simulink model "Jacobian"  (R2021a)
settings: Solver=FixedStepAuto  StartTime=0.0  StopTime=5  FixedStep=0.0001  RelTol=1e-3
libraries: aerolibutil x2
settings Model: Creator=negin  LastModifiedBy=negin

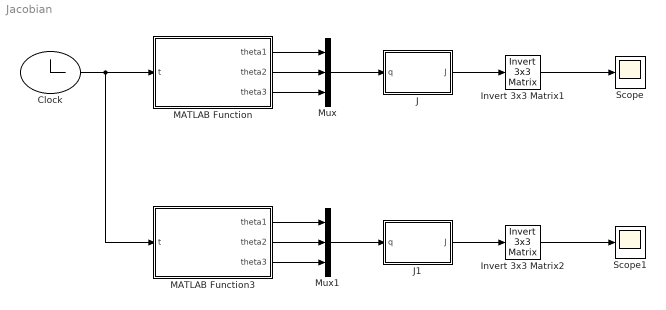
== system Jacobian ==
  Clock : Clock
  Invert 3x3 Matrix1 : aerolibutil/Invert  3x3 Matrix
  Invert 3x3 Matrix2 : aerolibutil/Invert  3x3 Matrix
  J : MATLAB Function  TreatAsAtomicUnit=on
  J1 : MATLAB Function  TreatAsAtomicUnit=on
  MATLAB Function : MATLAB Function  TreatAsAtomicUnit=on
  MATLAB Function3 : MATLAB Function  TreatAsAtomicUnit=on
  Mux : Mux  Inputs=3
  Mux1 : Mux  Inputs=3
  Scope : Scope
  Scope1 : Scope
  wires:
  Clock/1 -> MATLAB Function3/1(t), MATLAB Function/1(t)
  MATLAB Function/1(theta1) -> Mux/1
  MATLAB Function/2(theta2) -> Mux/2
  Mux/1 -> J/1(q)
  MATLAB Function/3(theta3) -> Mux/3
  J/1(J) -> Invert 3x3 Matrix1/1
  Invert 3x3 Matrix1/1 -> Scope/1
  J1/1(J) -> Invert 3x3 Matrix2/1
  Mux1/1 -> J1/1(q)
  MATLAB Function3/3(theta3) -> Mux1/3
  MATLAB Function3/2(theta2) -> Mux1/2
  MATLAB Function3/1(theta1) -> Mux1/1
  Invert 3x3 Matrix2/1 -> Scope1/1

== matlab function Jacobian/MATLAB Function ==
  data: theta1 output; t input; theta2 output; theta3 output
function [theta1, theta2, theta3] = desiredTraj(t)

% theta1 = 0.1309*t^2 + 0.0147*t^3 - 0.0085*t^4 + 0.0007*t^5;
% theta2 = 0.1309*t^2 - 0.0188*t^3 - 0.001*t^4 + 0.0002*t^5;
% theta3 = 0.1309*t^2 + 0.0314*t^3 - 0.0123*t^4 + 0.001*t^5;

theta1 = 2*exp(-0.1*t);
theta2 = 1 + exp(-0.15*t);
theta3 = 0.5 + 2*exp(-0.2*t);

end

== matlab function Jacobian/J ==
  data: J output; q input
function J = Jfun(q)

l1 = 1;
l2 = 1;
l3 = 1;

J11 = cos(q(1))*(l3*cos(q(2) + q(3)) + l2*cos(q(2)));
J12 = -sin(q(1))*(l3*sin(q(2) + q(3)) + l2*sin(q(2)));
J13 = -l3*sin(q(2) + q(3))*sin(q(1));
J21 = -sin(q(1))*(l3*cos(q(2) + q(3)) + l2*cos(q(2)));
J22 = -cos(q(1))*(l3*sin(q(2) + q(3)) + l2*sin(q(2)));
J23 = -l3*sin(q(2) + q(3))*cos(q(1));
J31 = 0;
J32 = l3*cos(q(2) + q(3)) + l2*cos(q(2));
J33 = l3*cos(q(2) + q(3));

J = [J11 J12 J13; J21 J22 J23; J31 J32 J33];

end

== matlab function Jacobian/J1 ==
  data: J output; q input
function J = Jfun(q)

l1 = 1;
l2 = 1;
l3 = 1;

J11 = cos(q(1))*(l3*cos(q(2) + q(3)) + l2*cos(q(2)));
J12 = -sin(q(1))*(l3*sin(q(2) + q(3)) + l2*sin(q(2)));
J13 = -l3*sin(q(2) + q(3))*sin(q(1));
J21 = -sin(q(1))*(l3*cos(q(2) + q(3)) + l2*cos(q(2)));
J22 = -cos(q(1))*(l3*sin(q(2) + q(3)) + l2*sin(q(2)));
J23 = -l3*sin(q(2) + q(3))*cos(q(1));
J31 = 0;
J32 = l3*cos(q(2) + q(3)) + l2*cos(q(2));
J33 = l3*cos(q(2) + q(3));

J = [J11 J12 J13; J21 J22 J23; J31 J32 J33];

end

== matlab function Jacobian/MATLAB Function3 ==
  data: theta1 output; t input; theta2 output; theta3 output
function [theta1, theta2, theta3] = desiredTraj(t)
theta1 = 0.1309*t^2 + 0.0147*t^3 - 0.0085*t^4 + 0.0007*t^5;
theta2 = 0.1309*t^2 - 0.0188*t^3 - 0.001*t^4 + 0.0002*t^5;
theta3 = 0.1309*t^2 + 0.0314*t^3 - 0.0123*t^4 + 0.001*t^5;
